simulink model "model"  (R2024b)
settings: Solver=VariableStepAuto  StartTime=0.0  StopTime=10.0  RelTol=1e-3
values from neighbouring files (symbols this model uses):
  C1 = M + Mu + (I_Gw / R^2)    (= 85.5001240002)    [init.m]    (also in state_var_model_kean.m = M + Mu + (I_Gw / R^2); test.m = M + Mu + (I_Gw / R^2))
  C2 = L_g * Mu    (= 50.5)    [init.m]    (also in state_var_model_kean.m = L_g * Mu; test.m = L_g * Mu)
  C4 = (Mu * L_g^2 + I_Gu)    (= 70.5)    [init.m]    (also in state_var_model_kean.m = (Mu * L_g^2 + I_Gu); test.m = (Mu * L_g^2 + I_Gu))
  g = 9.81    [init.m]
settings Model: Creator=sengu  LastModifiedBy=sengu

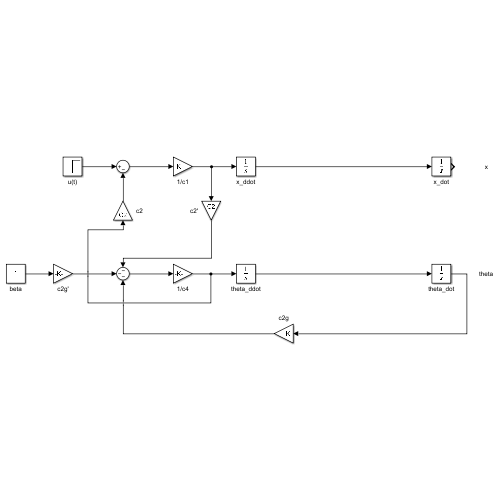
[thumbnail: Simulink's stored preview of the top-level diagram]
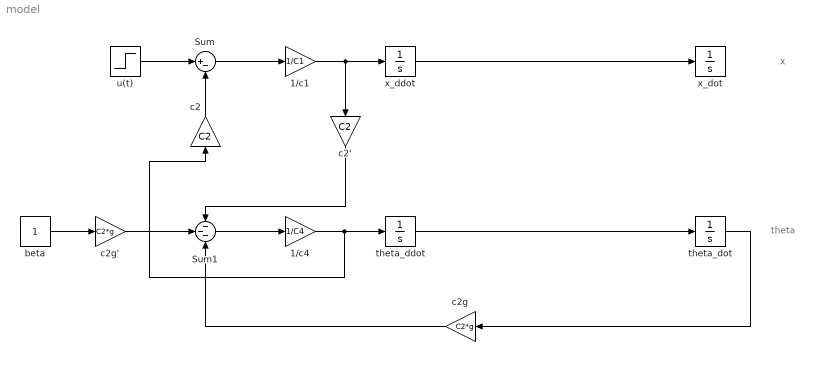
== system model ==
  note: theta
  note: x
  1/c1 : Gain  Gain=1/C1
  1/c4 : Gain  Gain=1/C4
  Sum : Sum  Inputs=|+-
  Sum1 : Sum  Inputs=---
  beta : Constant
  c2 : Gain  Gain=C2
  c2' : Gain  Gain=C2
  c2g : Gain  Gain=C2*g
  c2g' : Gain  Gain=C2*g
  theta_ddot : Integrator
  theta_dot : Integrator
  u(t) : Step  SampleTime=0
  x_ddot : Integrator
  x_dot : Integrator
  wires:
  1/c1/1 -> c2'/1, x_ddot/1
  Sum/1 -> 1/c1/1
  1/c4/1 -> c2/1, theta_ddot/1
  Sum1/1 -> 1/c4/1
  u(t)/1 -> Sum/1
  c2/1 -> Sum/2
  x_ddot/1 -> x_dot/1
  theta_ddot/1 -> theta_dot/1
  c2'/1 -> Sum1/1
  theta_dot/1 -> c2g/1
  c2g/1 -> Sum1/3
  beta/1 -> c2g'/1
  c2g'/1 -> Sum1/2
